simulink model "Autopilot"  (R2016a)
settings: Solver=FixedStepDiscrete  StartTime=0.0  StopTime=25  FixedStep=1/40  MaxStep=1/40  RelTol=1e-2  AbsTol=1e-3
PreLoadFcn:
  | Autopilot_bus;
model workspace (MAT data in the model file):
  beaver_init_roll = 0
  tmp20121902TempDataBlockParam11960188 = 1
  tmp20121902TempDataBlockParam15378051 = 1
  tmp20121902TempDataBlockParam16564336 = 1
  tmp2399823TempDataBlockParam27430435 = 11
  tmp2399823TempDataBlockParam30328219 = 20
  tmp2399823TempDataBlockParam8793363 = 1
undefined symbols (not defined in the file or in its folder): dispGain, hdgGain, intGain, rateGain
libraries: simulink x1
settings Model: ExtModeTrigMode=oneshot  ExtModeArmWhenConnect=off  ExtModeAutoUpdateStatusClock=off  Creator=The MathWorks Inc.  LastModifiedBy=ceren.gebizli
settings DataIOCC: ExternalInput=apin  LoadExternalInput=on  SaveFormat=StructureWithTime  DSMLogging=off  SignalLoggingName=sigsOut
settings OptimizationCC: BlockReduction=off  ConditionallyExecuteInputs=off  DefaultParameterBehavior=Inlined  InlineInvariantSignals=on  ExpressionDepthLimit=2147483647  InitFltsAndDblsToZero=on  EfficientFloat2IntCast=on  EfficientMapNaN2IntZero=off  OptimizeModelRefInitCode=on  MaxStackSize=inf
settings DebuggingCC: SignalInfNanChecking=error  SignalRangeChecking=error  ReadBeforeWriteMsg=EnableAllAsError  WriteAfterWriteMsg=EnableAllAsError  WriteAfterReadMsg=EnableAllAsError  AlgebraicLoopMsg=error  ArtificialAlgebraicLoopMsg=error  SaveWithDisabledLinksMsg=error  SaveWithParameterizedLinksMsg=error  CheckExecutionContextPreStartOutputMsg=on  CheckExecutionContextRuntimeOutputMsg=on  BlockPriorityViolationMsg=error  MaxConsecutiveZCsMsg=warning  SolverPrmCheckMsg=error  InheritedTsInSrcMsg=error  SigSpecEnsureSampleTimeMsg=error  CheckMatrixSingularityMsg=error  IntegerOverflowMsg=error  ParameterUnderflowMsg=error  ParameterPrecisionLossMsg=error  ParameterTunabilityLossMsg=error  UnderSpecifiedDataTypeMsg=error  UnnecessaryDatatypeConvMsg=warning  VectorMatrixConversionMsg=error  SignalLabelMismatchMsg=error  UnconnectedInputMsg=error  UnconnectedOutputMsg=error  UnconnectedLineMsg=error  SFcnCompatibilityMsg=error  BusObjectLabelMismatch=error  RootOutportRequireBusObject=error  AssertControl=DisableAll  ModelReferenceIOMsg=error  ModelReferenceIOMismatchMessage=error  UnknownTsInhSupMsg=error  ModelReferenceDataLoggingMessage=error  StateNameClashWarn=warning  StrictBusMsg=ErrorOnBusTreatedAsVector  NonBusSignalsTreatedAsBus=error  IntegerSaturationMsg=error
settings HardwareCC: ProdBitPerPointer=32  ProdLargestAtomicFloat=None  ProdEndianess=BigEndian  ProdWordSize=32  ProdHWDeviceType=32-bit Embedded Processor  TargetHWDeviceType=32-bit Generic
settings ModelReferenceCC: CheckModelReferenceTargetMessage=none  PropagateSignalLabelsOutOfModel=off
settings RTWCC: SystemTargetFile=ert.tlc  TemplateMakefile=ert_default_tmf  Description=Real-Time Workshop Embedded Coder (no auto configuration)  GenerateReport=on  RTWVerbose=off  IncludeHyperlinkInReport=on  LaunchReport=on  PortableWordSizes=on  GenerateTraceInfo=on  GenerateTraceReport=on  GenerateTraceReportSl=on  GenerateTraceReportSf=on  GenerateTraceReportEml=on
settings CodeAppCC: ForceParamTrailComments=on  IgnoreCustomStorageClasses=off  MaxIdLength=63  MangleLength=4  CustomSymbolStrType=$N$R$M  InternalIdentifier=Classic  ReqsInCode=on
settings ERTTargetCC: TargetFcnLib=ansi_tfl_tmw.mat  UtilityFuncGeneration=Shared location  GenerateSampleERTMain=on  IncludeMdlTerminateFcn=off  GeneratePreprocessorConditionals=Disable all  SuppressErrorStatus=on  SupportAbsoluteTime=off  SupportNonFinite=off  SupportComplex=off  ParenthesesLevel=Maximum  InlinedParameterPlacement=NonHierarchical  MultiInstanceErrorCode=None  ERTCustomFileTemplate=example_file_process.tlc  PreserveExpressionOrder=on  PreserveIfCondition=on  ConvertIfToSwitch=off  SuppressUnreachableDefaultCases=off
settings ConfigComp: CovMetricSettings=dcmtrzoiwe  CovHTMLOptions=-sRT=1 -aTS=1 -bRG=1 -bTC=1 -hTR=0 -nFC=0 -scm=1 -bcm=1 -xEv=0  CovHtmlReporting=off  CovSaveSingleToWorkspaceVar=off  CovCumulativeReport=on  CovReportOnPause=off  PSOpenProjectManager=on  PSSendToPolyspaceServer=on  PSModelRefVerifDepth=All  PSAutoStubLUT=off

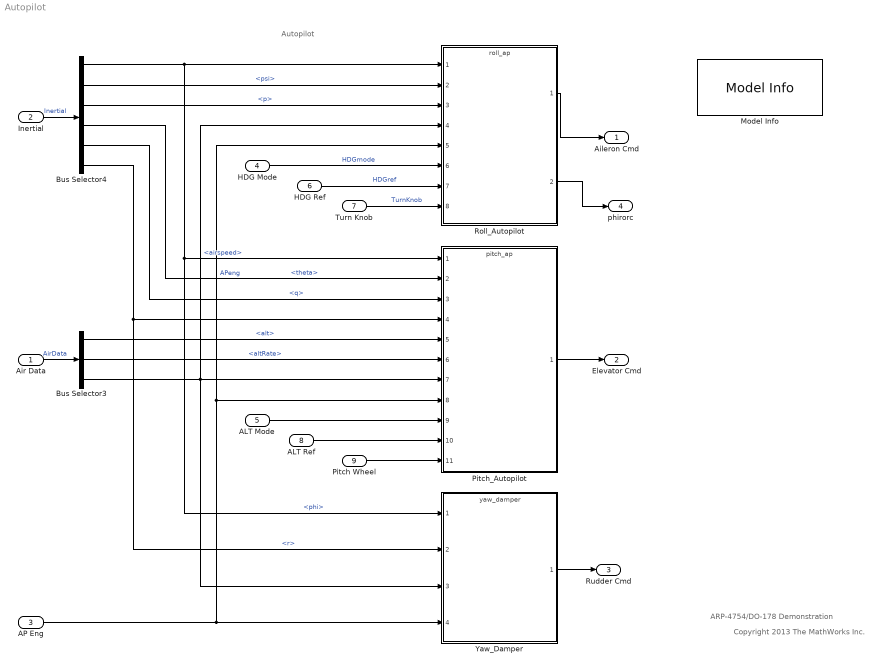
== system Autopilot ==
  note: Autopilot
  note: Copyright 2013 The MathWorks Inc.
  note: ARP-4754/DO-178 Demonstration
  Air Data : Inport  OutDataTypeStr=Bus: slBus1  SampleTime=[0.025000000000000001,0]  BusOutputAsStruct=on
  Inertial : Inport  Port=2  OutDataTypeStr=Bus: slBus2  SampleTime=[0.025000000000000001,0]  BusOutputAsStruct=on
  AP Eng : Inport  Port=3  OutMin=0  OutMax=1  OutDataTypeStr=boolean  PortDimensions=1  SampleTime=[0.025000000000000001,0]
  HDG Mode : Inport  Port=4  OutMin=0  OutMax=1  OutDataTypeStr=boolean  PortDimensions=1  SampleTime=[0.025000000000000001,0]
  ALT Mode : Inport  Port=5  OutMin=0  OutMax=1  OutDataTypeStr=boolean  PortDimensions=1  SampleTime=[0.025000000000000001,0]
  HDG Ref : Inport  Port=6  OutMin=-180  OutMax=180  OutDataTypeStr=double  PortDimensions=1  SampleTime=[0.025000000000000001,0]
  Turn Knob : Inport  Port=7  OutMin=-45  OutMax=45  OutDataTypeStr=double  PortDimensions=1  SampleTime=[0.025000000000000001,0]
  ALT Ref : Inport  Port=8  OutMin=0  OutMax=65000  OutDataTypeStr=double  PortDimensions=1  SampleTime=[0.025000000000000001,0]
  Pitch Wheel : Inport  Port=9  OutMin=-30  OutMax=30  OutDataTypeStr=double  PortDimensions=1  SampleTime=[0.025000000000000001,0]
  Bus Selector3 : BusSelector  OutputSignals=alt,altRate,airspeed
  Bus Selector4 : BusSelector  OutputSignals=phi,psi,p,theta,q,r
  Model Info : simulink/Model-Wide Utilities/Model Info  BlockCM=none  Frame=on  DisplayStringWithTags=|  HorizontalTextAlignment=Left  LeftAlignmentValue=0.02  SourceBlockDiagram=Autopilot  TagMaxNumber=20
      | Autopilot
      | Author: %<LastModifiedBy>
      | Date: %<LastModificationDate>
      | Model Version: %<ModelVersion>
  Pitch_Autopilot : ModelReference  ModelNameDialog=pitch_ap  ParameterArgumentNames=dispGain,intGain,rateGain  ParameterArgumentValues=2.0, 0.5, 2.0  SimulationMode=Normal  ModelReferenceVersion=1.90
  Roll_Autopilot : ModelReference  ModelNameDialog=roll_ap  ParameterArgumentNames=dispGain,intGain,rateGain,hdgGain  ParameterArgumentValues=1.0, 1.0, 3.0, 0.015  SimulationMode=Normal  ModelReferenceVersion=1.171
  Yaw_Damper : ModelReference  ModelNameDialog=yaw_damper  ParameterArgumentNames=rateGain  ParameterArgumentValues=1.0  SimulationMode=Normal  ModelReferenceVersion=1.80
  Aileron Cmd : Outport  OutDataTypeStr=double  PortDimensions=1  SampleTime=[0.025000000000000001,0]
  Elevator Cmd : Outport  Port=2  OutDataTypeStr=double  PortDimensions=1  SampleTime=[0.025000000000000001,0]
  Rudder Cmd : Outport  Port=3  OutDataTypeStr=double  PortDimensions=1  SampleTime=[0.025000000000000001,0]
  phirorc : Outport  Port=4  OutDataTypeStr=double  PortDimensions=1  SampleTime=[0.025000000000000001,0]
  wires:
  Bus Selector4/4 -> Pitch_Autopilot/2  "<theta>"
  Bus Selector4/5 -> Pitch_Autopilot/3  "<q>"
  Bus Selector4/6 -> Yaw_Damper/2, Pitch_Autopilot/4  "<r>"
  Air Data/1 -> Bus Selector3/1  "AirData"
  Inertial/1 -> Bus Selector4/1  "Inertial"
  Roll_Autopilot/1 -> Aileron Cmd/1
  HDG Mode/1 -> Roll_Autopilot/6  "HDGmode"
  HDG Ref/1 -> Roll_Autopilot/7  "HDGref"
  Turn Knob/1 -> Roll_Autopilot/8  "TurnKnob"
  Bus Selector4/3 -> Roll_Autopilot/3  "<p>"
  Bus Selector4/2 -> Roll_Autopilot/2  "<psi>"
  Bus Selector4/1 -> Roll_Autopilot/1, Pitch_Autopilot/1, Yaw_Damper/1  "<phi>"
  ALT Mode/1 -> Pitch_Autopilot/9
  Bus Selector3/3 -> Pitch_Autopilot/7, Roll_Autopilot/4, Yaw_Damper/3  "<airspeed>"
  Bus Selector3/2 -> Pitch_Autopilot/6  "<altRate>"
  ALT Ref/1 -> Pitch_Autopilot/10
  Pitch Wheel/1 -> Pitch_Autopilot/11
  Pitch_Autopilot/1 -> Elevator Cmd/1
  Bus Selector3/1 -> Pitch_Autopilot/5  "<alt>"
  AP Eng/1 -> Yaw_Damper/4, Pitch_Autopilot/8, Roll_Autopilot/5  "APeng"
  Yaw_Damper/1 -> Rudder Cmd/1
  Roll_Autopilot/2 -> phirorc/1
